simulink model "condiciones_iniciales_model"  (R2020a)
settings: Solver=VariableStepAuto  StartTime=0.0  StopTime=300  RelTol=1e-3
values from neighbouring files (symbols this model uses):
  bp = 0.05    [simulacion.m]
  kp = 3.0    (= 3)    [simulacion.m]
  kp_poc = 0.4    [simulacion.m]
  SP1 = 180    [simulacion.m]
  t3 = 0.01    [simulacion.m]
  td = 0    [simulacion.m]
  tn_poc = 5    [simulacion.m]
  tx = 0.8    [simulacion.m]
libraries: simulink x2
settings Model: Creator=Lenovo  LastModifiedBy=Lenovo

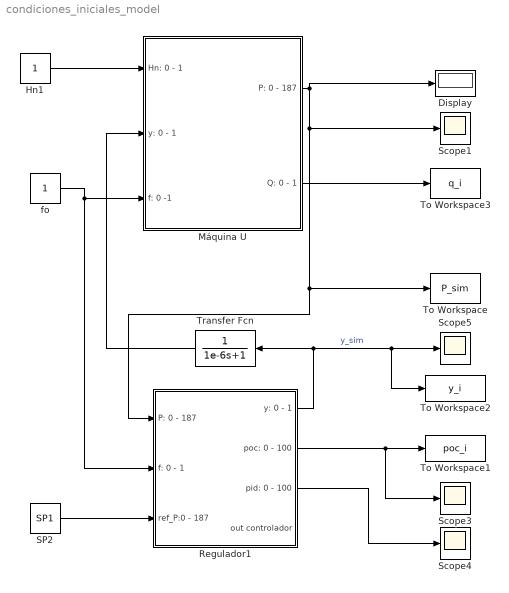
== system condiciones_iniciales_model ==
  Display : Display
  Hn1 : Constant
  Máquina U : Subsystem
  Regulador1 : Subsystem
  SP2 : Constant  Value=SP1
  Scope{1,3..5} (4 alike) : Scope
  To Workspace : ToWorkspace  VariableName=P_sim  SaveFormat=Timeseries  SampleTime=1
  To Workspace1 : ToWorkspace  VariableName=poc_i  SampleTime=-1
      settings: MaxDataPoints=1
  To Workspace2 : ToWorkspace  VariableName=y_i  SampleTime=-1
      settings: MaxDataPoints=1
  To Workspace3 : ToWorkspace  VariableName=q_i  SampleTime=1
      settings: MaxDataPoints=1
  Transfer Fcn : TransferFcn  Denominator=[1e-6 1]
  fo : Constant
  wires:
  Regulador1/3(pid: 0 - 100) -> Scope4/1
  fo/1 -> Máquina U/3(f: 0 -1), Regulador1/2(f: 0 - 1)
  Hn1/1 -> Máquina U/1(Hn: 0 - 1)
  Regulador1/1(y: 0 - 1) -> To Workspace2/1, Scope5/1, Transfer Fcn/1  "y_sim"
  Máquina U/1(P: 0 - 187) -> Display/1, Scope1/1, Regulador1/1(P: 0 - 187), To Workspace/1
  SP2/1 -> Regulador1/3(ref_P:0 - 187)
  Regulador1/2(poc: 0 - 100) -> To Workspace1/1, Scope3/1
  Transfer Fcn/1 -> Máquina U/2(y: 0 - 1)
  Máquina U/2(Q: 0 - 1) -> To Workspace3/1

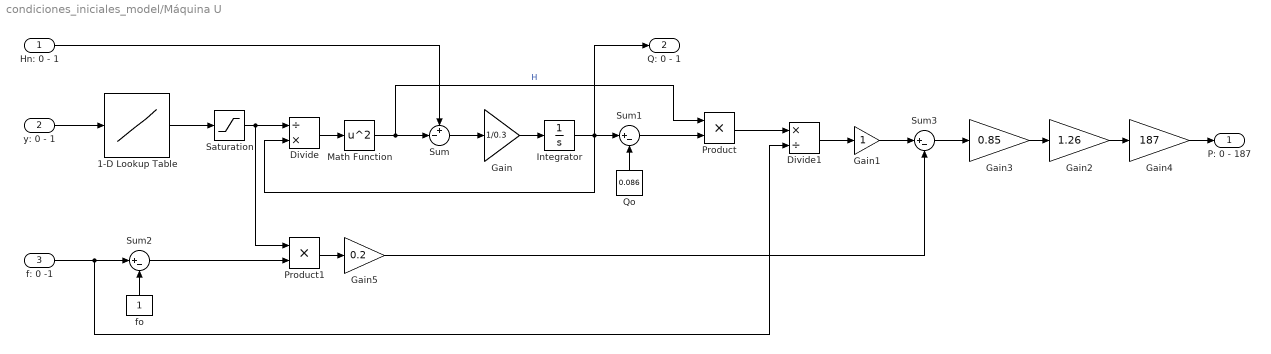
== system condiciones_iniciales_model/Máquina U ==
  Hn: 0 - 1 : Inport
  y: 0 - 1 : Inport  Port=2
  f: 0 -1 : Inport  Port=3
  1-D Lookup Table : Lookup_n-D  NumberOfTableDimensions=1  BreakpointsForDimension1=[0,0.072,0.336,0.35,0.4,0.45,0.5,0.55,0.6,0.65,0.7,0.75,0.8,0.85,0.9,0.95,1]  Table=[0,0.086,0.387,0.4035,0.4592,0.5194,0.5826,0.6475,0.7127,0.777,0.8389,0.8971,0.9502,0.9969,1.0358,1.0656,1.0849]  InternalRulePriority=Speed  RndMeth=Simplest  InputSameDT=on
  Divide : Product  Inputs=/*
  Divide1 : Product  Inputs=*/
  Gain : Gain  Gain=1/0.3
  Gain1 : Gain
  Gain2 : Gain  Gain=1.26
  Gain3 : Gain  Gain=0.85
  Gain4 : Gain  Gain=187
  Gain5 : Gain  Gain=0.2
  Integrator : Integrator  InitialCondition=0.3
  Math Function : Math  Operator=square  SaturateOnIntegerOverflow=on
  Product : Product
  Product1 : Product
  Qo : Constant  Value=0.086
  Saturation : Saturate  UpperLimit=1.1  LowerLimit=0.0001
  Sum : Sum  Inputs=+-|
  Sum1 : Sum  Inputs=|+-
  Sum2 : Sum  Inputs=|+-
  Sum3 : Sum  Inputs=|+-
  fo : Constant
  P: 0 - 187 : Outport
  Q: 0 - 1 : Outport  Port=2
  wires:
  Math Function/1 -> Sum/2, Product/1  "H"
  Integrator/1 -> Q: 0 - 1/1, Sum1/1, Divide/2
  Qo/1 -> Sum1/2
  Gain2/1 -> Gain4/1
  y: 0 - 1/1 -> 1-D Lookup Table/1
  Saturation/1 -> Divide/1, Product1/1
  1-D Lookup Table/1 -> Saturation/1
  f: 0 -1/1 -> Divide1/2, Sum2/1
  Gain1/1 -> Sum3/1
  Sum1/1 -> Product/2
  Product1/1 -> Gain5/1
  Divide1/1 -> Gain1/1
  Sum2/1 -> Product1/2
  Divide/1 -> Math Function/1
  Product/1 -> Divide1/1
  Hn: 0 - 1/1 -> Sum/1
  Gain5/1 -> Sum3/2
  Sum3/1 -> Gain3/1
  Sum/1 -> Gain/1
  Gain/1 -> Integrator/1
  Gain3/1 -> Gain2/1
  fo/1 -> Sum2/2
  Gain4/1 -> P: 0 - 187/1

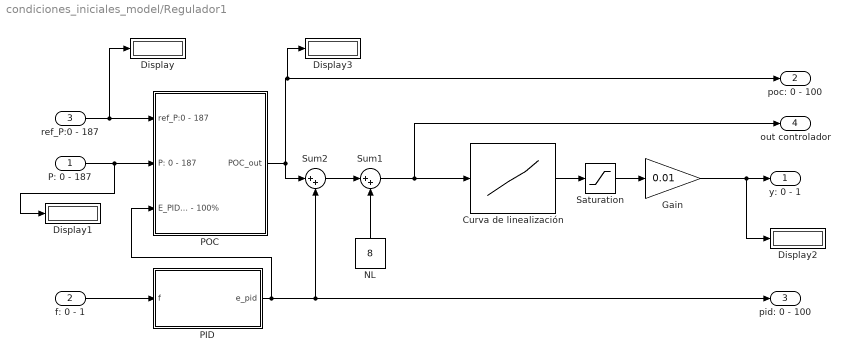
== system condiciones_iniciales_model/Regulador1 ==
  P: 0 - 187 : Inport
  f: 0 - 1 : Inport  Port=2
  ref_P:0 - 187 : Inport  Port=3
  Curva de linealización : Lookup_n-D  NumberOfTableDimensions=1  BreakpointsForDimension1=[-1,0,8,8.001,18,38,48,58,68,78,88,98,107,151]  Table=[-1,0,8,8.001,17.4,33.1,40,46.3,51.8,59.0,67,78,89,115]  InternalRulePriority=Speed  RndMeth=Simplest  InputSameDT=on
  Display{,1..3} (4 alike) : Display
  Gain : Gain  Gain=0.01
  NL : Constant  Value=8
  PID : Subsystem
  POC : Subsystem
  Saturation : Saturate  UpperLimit=115  LowerLimit=7.9  ZeroCross=off
  Sum1 : Sum  Inputs=|++
  Sum2 : Sum  Inputs=|++
  y: 0 - 1 : Outport
  poc: 0 - 100 : Outport  Port=2
  pid: 0 - 100 : Outport  Port=3
  out controlador : Outport  Port=4
  wires:
  PID/1(e_pid) -> POC/3(E_PID: 0 - 100%), Sum2/2, pid: 0 - 100/1
  POC/1(POC_out) -> Display3/1, poc: 0 - 100/1, Sum2/1
  f: 0 - 1/1 -> PID/1(f)
  NL/1 -> Sum1/2
  Sum2/1 -> Sum1/1
  ref_P:0 - 187/1 -> Display/1, POC/1(ref_P:0 - 187)
  P: 0 - 187/1 -> Display1/1, POC/2(P: 0 - 187)
  Saturation/1 -> Gain/1
  Curva de linealización/1 -> Saturation/1
  Gain/1 -> Display2/1, y: 0 - 1/1
  Sum1/1 -> out controlador/1, Curva de linealización/1

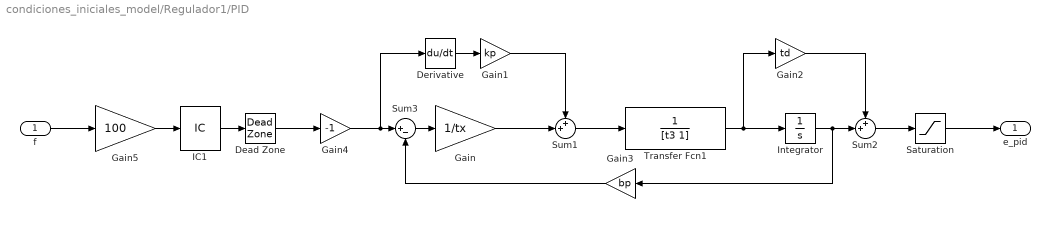
== system condiciones_iniciales_model/Regulador1/PID ==
  f : Inport
  Dead Zone : DeadZone  LowerValue=100-0.01  UpperValue=100+0.01  SaturateOnIntegerOverflow=on
  Derivative : Derivative
  Gain : Gain  Gain=1/tx
  Gain1 : Gain  Gain=kp
  Gain2 : Gain  Gain=td
  Gain3 : Gain  Gain=bp
  Gain4 : Gain  Gain=-1
  Gain5 : Gain  Gain=100
  IC1 : InitialCondition  Value=100
  Integrator : Integrator
  Saturation : Saturate  UpperLimit=2.5  LowerLimit=-2.5
  Sum1 : Sum  Inputs=++|
  Sum2 : Sum  Inputs=++|
  Sum3 : Sum  Inputs=|+-
  Transfer Fcn1 : TransferFcn  Denominator=[t3 1]
  e_pid : Outport
  wires:
  Saturation/1 -> e_pid/1
  Transfer Fcn1/1 -> Integrator/1, Gain2/1
  Gain2/1 -> Sum2/1
  Sum1/1 -> Transfer Fcn1/1
  Dead Zone/1 -> Gain4/1
  Integrator/1 -> Sum2/2, Gain3/1
  Gain3/1 -> Sum3/2
  f/1 -> Gain5/1
  Derivative/1 -> Gain1/1
  IC1/1 -> Dead Zone/1
  Gain4/1 -> Sum3/1, Derivative/1
  Gain/1 -> Sum1/2
  Gain1/1 -> Sum1/1
  Sum2/1 -> Saturation/1
  Sum3/1 -> Gain/1
  Gain5/1 -> IC1/1

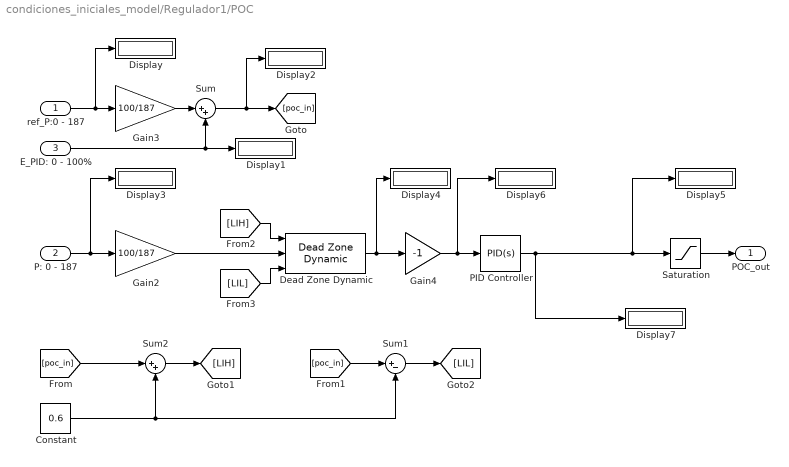
== system condiciones_iniciales_model/Regulador1/POC ==
  ref_P:0 - 187 : Inport
  P: 0 - 187 : Inport  Port=2
  E_PID: 0 - 100% : Inport  Port=3
  Constant : Constant  Value=0.6
  Dead Zone Dynamic : simulink/Discontinuities/Dead Zone Dynamic
      settings: SourceProductBaseCode=SL
  Display{,1..7} (8 alike) : Display
  Gain2 : Gain  Gain=100/187
  Gain3 : Gain  Gain=100/187
  Gain4 : Gain  Gain=-1
  PID Controller : simulink/Continuous/PID Controller  Controller=PID  Form=Parallel  TimeDomain=Continuous-time  UseExternalTs=off  SampleTime=-1  IntegratorMethod=Forward Euler  FilterMethod=Forward Euler  ControllerParametersSource=internal  P=kp_poc  I=kp_poc/tn_poc  D=0  UseFilter=on  N=100  TunerSelectOption=Transfer Function Based (PID Tuner App)  InitialConditionSource=internal  InitialConditionForIntegrator=0  InitialConditionForFilter=0  DifferentiatorICPrevScaledInput=0  ExternalReset=none  TrackingMode=off  Kt=1  LimitOutput=off  UpperSaturationLimit=inf  LowerSaturationLimit=-inf  LinearizeAsGain=on  AntiWindupMode=none  Kb=1  POutMin=[]  POutMax=[]  IOutMin=[]  IOutMax=[]  DOutMin=[]  DOutMax=[]  NOutMin=[]  NOutMax=[]  SumOutMin=[]  SumOutMax=[]  SaturationOutMin=[]  SaturationOutMax=[]  PParamMin=[]  PParamMax=[]  IParamMin=[]  IParamMax=[]  DParamMin=[]  DParamMax=[]  NParamMin=[]  NParamMax=[]  KbParamMin=[]  KbParamMax=[]  KtParamMin=[]  KtParamMax=[]  KbOutMin=[]  KbOutMax=[]  KtOutMin=[]  KtOutMax=[]  IntegratorOutMin=[]  IntegratorOutMax=[]  FilterOutMin=[]  FilterOutMax=[]  SumI1OutMin=[]  SumI1OutMax=[]  SumI2OutMin=[]  SumI2OutMax=[]  SumI3OutMin=[]  SumI3OutMax=[]  SumI4OutMin=[]  SumI4OutMax=[]  SumDOutMin=[]  SumDOutMax=[]  DifferentiatorOutMin=[]  DifferentiatorOutMax=[]  FilterDiffOutCoefMin=[]  FilterDiffOutCoefMax=[]  ReciprocalOutMin=[]  ReciprocalOutMax=[]  SumDenOutMin=[]  SumDenOutMax=[]  SumNumOutMin=[]  SumNumOutMax=[]  DivideOutMin=[]  DivideOutMax=[]  UdiffTsProdOutMin=[]  UdiffTsProdOutMax=[]  NTsProdOutMin=[]  NTsProdOutMax=[]  UintegralTsProdOutMin=[]  UintegralTsProdOutMax=[]  UngainTsProdOutMin=[]  UngainTsProdOutMax=[]  IntegratorContinuousStateAttributes=''  IntegratorStateMustResolveToSignalObject=off  IntegratorRTWStateStorageClass=Auto  FilterContinuousStateAttributes=''  FilterStateMustResolveToSignalObject=off  FilterRTWStateStorageClass=Auto  ParallelPVariant=InternalParameters  IdealPVariant=Disabled  IVariant=InternalParameters  DVariant=InternalParameters  IntegratorVariant=Continuous  SatVariant=Disabled  AWVariant=Passthrough  PCopyVariant=Disabled  TRVariant=Disabled  FdbkBlocksVariant=Forward  IdealPFdbkVariant=Disabled  SatFdbkVariant=Disabled  DerivativeFilterVariant=ContFilter  NVariant=InternalParameters  NCopyVariant=Disabled  FilterICVariant=InternalICsFilter  IntegratorICVariant=InternalICs  ExternalResetVariant=Disabled  TRSumVariant=Passthrough  SumFdbkVariant=Disabled  SumVariant=Sum_PID  TsampFilterVariant=InternalTs  TsampNgainVariant=Passthrough  TsampIntegralVariant=Passthrough
  Saturation : Saturate  UpperLimit=120  LowerLimit=-1  ZeroCross=off
  Sum : Sum  Inputs=|++
  Sum1 : Sum  Inputs=|+-
  Sum2 : Sum  Inputs=|++
  POC_out : Outport
  wires:
  Sum2/1 -> [LIH]
  [LIL] -> Dead Zone Dynamic/3
  Gain3/1 -> Sum/1
  [poc_in] -> Sum1/1
  Sum1/1 -> [LIL]
  PID Controller/1 -> Display5/1, Saturation/1, Display7/1
  Gain4/1 -> Display6/1, PID Controller/1
  Dead Zone Dynamic/1 -> Display4/1, Gain4/1
  E_PID: 0 - 100%/1 -> Display1/1, Sum/2
  ref_P:0 - 187/1 -> Display/1, Gain3/1
  [LIH] -> Dead Zone Dynamic/1
  Saturation/1 -> POC_out/1
  Sum/1 -> Display2/1, [poc_in]
  Gain2/1 -> Dead Zone Dynamic/2
  Constant/1 -> Sum2/2, Sum1/2
  [poc_in] -> Sum2/1
  P: 0 - 187/1 -> Display3/1, Gain2/1
